simulink model "sm_car_display_battery_model"  (R2021a)
settings: Solver=VariableStepAuto  StartTime=0.0  StopTime=10.0  RelTol=1e-3
undefined symbols (not defined in the file or in its folder): X, Y, Z
libraries: sm_lib x98, nesl_utility x72, Cooling_Components x1
(part 4 of 4)

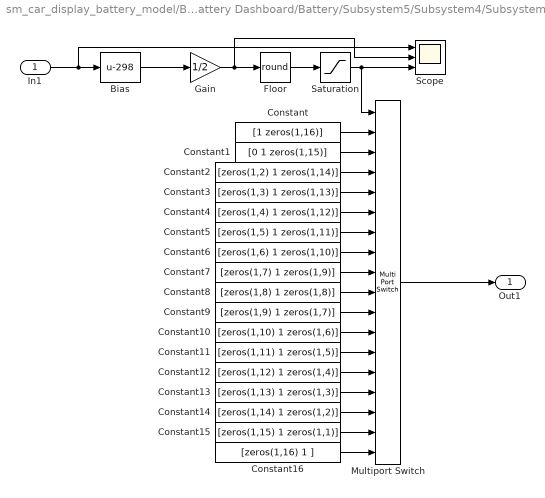
== system sm_car_display_battery_model/Battery Dashboard/Battery/Subsystem5/Subsystem4/Subsystem3 ==
  In1 : Inport
  Bias : Bias  Bias=-298
  Constant : Constant  Value=[1 zeros(1,16)]
  Constant1 : Constant  Value=[0 1 zeros(1,15)]
  Constant10 : Constant  Value=[zeros(1,10) 1 zeros(1,6)]
  Constant11 : Constant  Value=[zeros(1,11) 1 zeros(1,5)]
  Constant12 : Constant  Value=[zeros(1,12) 1 zeros(1,4)]
  Constant13 : Constant  Value=[zeros(1,13) 1 zeros(1,3)]
  Constant14 : Constant  Value=[zeros(1,14) 1 zeros(1,2)]
  Constant15 : Constant  Value=[zeros(1,15) 1 zeros(1,1)]
  Constant16 : Constant  Value=[zeros(1,16) 1 ]
  Constant2 : Constant  Value=[zeros(1,2) 1 zeros(1,14)]
  Constant3 : Constant  Value=[zeros(1,3) 1 zeros(1,13)]
  Constant4 : Constant  Value=[zeros(1,4) 1 zeros(1,12)]
  Constant5 : Constant  Value=[zeros(1,5) 1 zeros(1,11)]
  Constant6 : Constant  Value=[zeros(1,6) 1 zeros(1,10)]
  Constant7 : Constant  Value=[zeros(1,7) 1 zeros(1,9)]
  Constant8 : Constant  Value=[zeros(1,8) 1 zeros(1,8)]
  Constant9 : Constant  Value=[zeros(1,9) 1 zeros(1,7)]
  Floor : Rounding  Operator=round
  Gain : Gain  Gain=1/2
  Multiport Switch : MultiPortSwitch  DataPortOrder=Zero-based contiguous  Inputs=17  zeroidx=on
  Saturation : Saturate  UpperLimit=16  LowerLimit=0
  Scope : Scope  NumInputPorts=3
  Out1 : Outport  VectorParamsAs1DForOutWhenUnconnected=off
  wires:
  Saturation/1 -> Scope/3, Multiport Switch/1
  Constant9/1 -> Multiport Switch/11
  Constant12/1 -> Multiport Switch/14
  Constant1/1 -> Multiport Switch/3
  Constant13/1 -> Multiport Switch/15
  Constant8/1 -> Multiport Switch/10
  Constant7/1 -> Multiport Switch/9
  Constant4/1 -> Multiport Switch/6
  Constant5/1 -> Multiport Switch/7
  Bias/1 -> Gain/1
  Constant/1 -> Multiport Switch/2
  Constant15/1 -> Multiport Switch/17
  In1/1 -> Bias/1, Scope/1
  Constant6/1 -> Multiport Switch/8
  Multiport Switch/1 -> Out1/1
  Constant10/1 -> Multiport Switch/12
  Constant14/1 -> Multiport Switch/16
  Gain/1 -> Floor/1, Scope/2
  Constant2/1 -> Multiport Switch/4
  Floor/1 -> Saturation/1
  Constant11/1 -> Multiport Switch/13
  Constant16/1 -> Multiport Switch/18
  Constant3/1 -> Multiport Switch/5

== matlab function sm_car_display_battery_model/Battery Dashboard/Cooling Indicator/MATLAB Function1 ==
  data: AC input; AC_on output; AC_off output
function [AC_on,AC_off]= fcn(AC)

if AC > 0 
    AC_on = 1;
    AC_off = 0.001;
    
else
    AC_off = 1;
    AC_on = 0.001;
end
